simulink model "arte"  (R2013b)
(part 2 of 43)

  post_fft_delay1/3(Out2) -> antenna_power1/3(din1), [fft1_1]
  post_fft_delay1/4(Out3) -> antenna_power1/4(din2), [fft1_2]
  post_fft_delay1/5(Out4) -> antenna_power1/5(din3), [fft1_3]
  asiaa_adc5g0/12(c3) -> conv_bus1/5(i3)
  asiaa_adc5g0/14(c5) -> conv_bus1/7(i5)
  asiaa_adc5g0/10(c1) -> conv_bus1/3(i1)
  asiaa_adc5g0/13(c4) -> conv_bus1/6(i4)
  asiaa_adc5g0/9(c0) -> conv_bus1/2(i0)
  asiaa_adc5g0/15(c6) -> conv_bus1/8(i6)
  asiaa_adc5g0/16(c7) -> conv_bus1/9(i7)
  asiaa_adc5g0/11(c2) -> conv_bus1/4(i2)
  Black Box2/6 -> Terminator4/1
  bus_create2/1(bus_out) -> pipeline44/1
  pipeline44/1 -> adcsnap2/1(din)
  [cnt_rst] -> acc_cntrl2/3(rst)
  [acc_len] -> acc_cntrl2/1(acc_len)
  simple_bram_vacc_0_8/1(dout) -> pre_bram_delay2/2(In1)
  pipeline104/1(q) -> simple_bram_vacc_0_8/2(din)
  pipeline50/1(q) -> pre_bram_delay2/1(sync_in)
  pipeline49/1(q) -> simple_bram_vacc_0_8/1(new_acc)
  simple_bram_vacc_0_9/1(dout) -> pre_bram_delay2/3(In2)
  pipeline52/1(q) -> simple_bram_vacc_0_9/2(din)
  pipeline55/1(q) -> simple_bram_vacc_0_9/1(new_acc)
  simple_bram_vacc_0_10/1(dout) -> pre_bram_delay2/4(In3)
  pipeline94/1(q) -> simple_bram_vacc_0_10/2(din)
  pipeline97/1(q) -> simple_bram_vacc_0_10/1(new_acc)
  simple_bram_vacc_0_11/1(dout) -> pre_bram_delay2/5(In4)
  simple_bram_vacc_0_11/2(valid) -> pre_bram_delay2/6(valid_in)
  pipeline98/1(q) -> simple_bram_vacc_0_11/2(din)
  pipeline102/1(q) -> simple_bram_vacc_0_11/1(new_acc)
  Delay43/1 -> pipeline104/1(d)
  Delay45/1 -> pipeline52/1(d)
  Delay46/1 -> pipeline94/1(d)
  Delay47/1 -> pipeline98/1(d)
  acc_cntrl2/1(new_acc) -> pipeline102/1(d), pipeline97/1(d), pipeline55/1(d), pipeline49/1(d), pipeline50/1(d)
  Black Box3/6 -> Terminator18/1
  [cnt_rst] -> acc_cntrl3/3(rst)
  [acc_len] -> acc_cntrl3/1(acc_len)
  simple_bram_vacc_0_12/1(dout) -> pre_bram_delay3/2(In1)
  pipeline123/1(q) -> simple_bram_vacc_0_12/2(din)
  pipeline108/1(q) -> pre_bram_delay3/1(sync_in)
  pre_bram_delay3/2(Out1) -> Reinterpret12/1
  pre_bram_delay3/6(valid_out) -> Counter4/2, antenna_3/3(we)
  pre_bram_delay3/1(sync_out) -> Counter4/1
  pipeline107/1(q) -> simple_bram_vacc_0_12/1(new_acc)
  simple_bram_vacc_0_13/1(dout) -> pre_bram_delay3/3(In2)
  pipeline109/1(q) -> simple_bram_vacc_0_13/2(din)
  pre_bram_delay3/3(Out2) -> Reinterpret5/1
  pipeline112/1(q) -> simple_bram_vacc_0_13/1(new_acc)
  simple_bram_vacc_0_14/1(dout) -> pre_bram_delay3/4(In3)
  pipeline113/1(q) -> simple_bram_vacc_0_14/2(din)
  pre_bram_delay3/4(Out3) -> Reinterpret6/1
  pipeline116/1(q) -> simple_bram_vacc_0_14/1(new_acc)
  simple_bram_vacc_0_15/1(dout) -> pre_bram_delay3/5(In4)
  simple_bram_vacc_0_15/2(valid) -> pre_bram_delay3/6(valid_in)
  pipeline117/1(q) -> simple_bram_vacc_0_15/2(din)
  pre_bram_delay3/5(Out4) -> Reinterpret10/1
  pipeline120/1(q) -> simple_bram_vacc_0_15/1(new_acc)
  Delay50/1 -> pipeline123/1(d)
  Delay51/1 -> pipeline109/1(d)
  Delay52/1 -> pipeline113/1(d)
  Delay1/1 -> pipeline117/1(d)
  acc_cntrl3/1(new_acc) -> pipeline108/1(d), pipeline120/1(d), pipeline116/1(d), pipeline112/1(d), pipeline107/1(d)
  antenna_power0/2(dout0) -> power_convert0/1(In1)
  antenna_power0/3(dout1) -> power_convert0/2(In2)
  antenna_power0/4(dout2) -> power_convert0/3(In3)
  antenna_power0/5(dout3) -> power_convert0/4(In4)
  antenna_power0/1(sync_out) -> pipeline127/1(d)
  antenna_power1/2(dout0) -> power_convert1/1(In1)
  antenna_power1/3(dout1) -> power_convert1/2(In2)
  antenna_power1/4(dout2) -> power_convert1/3(In3)
  antenna_power1/5(dout3) -> power_convert1/4(In4)
  antenna_power2/2(dout0) -> power_convert2/1(In1)
  antenna_power2/3(dout1) -> power_convert2/2(In2)
  antenna_power2/4(dout2) -> power_convert2/3(In3)
  antenna_power2/5(dout3) -> power_convert2/4(In4)
  antenna_power3/2(dout0) -> power_convert3/1(In1)
  antenna_power3/3(dout1) -> power_convert3/2(In2)
  antenna_power3/4(dout2) -> power_convert3/3(In3)
  antenna_power3/5(dout3) -> power_convert3/4(In4)
  antenna_power1/1(sync_out) -> pipeline128/1(d)
  antenna_power2/1(sync_out) -> pipeline129/1(d)
  antenna_power3/1(sync_out) -> pipeline130/1(d)
  Band-Limited White Noise1/1 -> asiaa_adc5g1/1(sim_a)
  Constant2/1 -> asiaa_adc5g1/3(sim_sync)
  Band-Limited White Noise3/1 -> asiaa_adc5g1/2(sim_c)
  asiaa_adc5g1/17(sync_out) -> Terminator2/1
  asiaa_adc5g1/1(a0) -> conv_bus2/2(i0)
  asiaa_adc5g1/2(a1) -> conv_bus2/3(i1)
  asiaa_adc5g1/3(a2) -> conv_bus2/4(i2)
  asiaa_adc5g1/4(a3) -> conv_bus2/5(i3)
  asiaa_adc5g1/5(a4) -> conv_bus2/6(i4)
  asiaa_adc5g1/6(a5) -> conv_bus2/7(i5)
  asiaa_adc5g1/7(a6) -> conv_bus2/8(i6)
  asiaa_adc5g1/8(a7) -> conv_bus2/9(i7)
  asiaa_adc5g1/12(c3) -> Subsystem/4(In4)
  asiaa_adc5g1/14(c5) -> Subsystem/6(In6)
  asiaa_adc5g1/10(c1) -> Subsystem/2(In2)
  asiaa_adc5g1/13(c4) -> Subsystem/5(In5)
  asiaa_adc5g1/9(c0) -> Subsystem/1(In1)
  asiaa_adc5g1/15(c6) -> Subsystem/7(In7)
  asiaa_adc5g1/16(c7) -> Subsystem/8(In8)
  asiaa_adc5g1/11(c2) -> Subsystem/3(In3)
  [sync_out] -> delay_wideband_prog0/1(sync)
  [sync_out] -> delay_wideband_prog1/1(sync)
  [sync_out] -> delay_wideband_prog2/1(sync)
  [sync_out] -> pipeline/1(d)
  [snap_trig] -> adcsnap0/2(we), adcsnap0/3(trig)
  [snap_trig] -> adcsnap1/2(we), adcsnap1/3(trig)
  [snap_trig] -> adcsnap2/2(we), adcsnap2/3(trig)
  [adc0_delay] -> delay_wideband_prog0/2(delay)
  [adc1_delay] -> delay_wideband_prog1/2(delay)
  [adc2_delay] -> delay_wideband_prog2/2(delay)
  Constant8/1 -> delay_wideband_prog0/3(ld_delay)
  Constant9/1 -> delay_wideband_prog1/3(ld_delay)
  Constant11/1 -> delay_wideband_prog2/3(ld_delay)
  delay_wideband_prog0/9(data_out7) -> pre_pfb_delay1/9(In1)
  delay_wideband_prog0/7(data_out5) -> pre_pfb_delay1/7(In8)
  delay_wideband_prog0/2(data_out0) -> pre_pfb_delay1/2(In3)
  delay_wideband_prog0/3(data_out1) -> pre_pfb_delay1/3(In4)
  delay_wideband_prog0/5(data_out3) -> pre_pfb_delay1/5(In6)
  delay_wideband_prog0/8(data_out6) -> pre_pfb_delay1/8(In9)
  delay_wideband_prog0/4(data_out2) -> pre_pfb_delay1/4(In5)
  delay_wideband_prog0/6(data_out4) -> pre_pfb_delay1/6(In7)
  delay_wideband_prog0/1(sync_out) -> pre_pfb_delay1/1(sync_in)
  delay_wideband_prog1/1(sync_out) -> pre_pfb_delay2/1(sync_in)
  delay_wideband_prog1/2(data_out0) -> pre_pfb_delay2/2(In3)
  delay_wideband_prog1/3(data_out1) -> pre_pfb_delay2/3(In4)
  delay_wideband_prog1/4(data_out2) -> pre_pfb_delay2/4(In5)
  delay_wideband_prog1/5(data_out3) -> pre_pfb_delay2/5(In6)
  delay_wideband_prog1/6(data_out4) -> pre_pfb_delay2/6(In7)
  delay_wideband_prog1/7(data_out5) -> pre_pfb_delay2/7(In8)
  delay_wideband_prog1/8(data_out6) -> pre_pfb_delay2/8(In9)
  delay_wideband_prog1/9(data_out7) -> pre_pfb_delay2/9(In1)
  delay_wideband_prog2/1(sync_out) -> pre_pfb_delay3/1(sync_in)
  delay_wideband_prog2/2(data_out0) -> pre_pfb_delay3/2(In3)
  delay_wideband_prog2/3(data_out1) -> pre_pfb_delay3/3(In4)
  delay_wideband_prog2/4(data_out2) -> pre_pfb_delay3/4(In5)
  delay_wideband_prog2/5(data_out3) -> pre_pfb_delay3/5(In6)
  delay_wideband_prog2/6(data_out4) -> pre_pfb_delay3/6(In7)
  delay_wideband_prog2/7(data_out5) -> pre_pfb_delay3/7(In8)
  delay_wideband_prog2/8(data_out6) -> pre_pfb_delay3/8(In9)
  delay_wideband_prog2/9(data_out7) -> pre_pfb_delay3/9(In1)
  conv_bus4/1(q0) -> delay_wideband_prog0/4(data_in0)
  conv_bus4/2(q1) -> delay_wideband_prog0/5(data_in1)
  conv_bus4/3(q2) -> delay_wideband_prog0/6(data_in2)
  conv_bus4/4(q3) -> delay_wideband_prog0/7(data_in3)
  conv_bus4/5(q4) -> delay_wideband_prog0/8(data_in4)
  conv_bus4/6(q5) -> delay_wideband_prog0/9(data_in5)
  conv_bus4/7(q6) -> delay_wideband_prog0/10(data_in6)
  conv_bus4/8(q7) -> delay_wideband_prog0/11(data_in7)
  conv_bus1/1(q0) -> delay_wideband_prog1/4(data_in0)
  conv_bus1/2(q1) -> delay_wideband_prog1/5(data_in1)
  conv_bus1/3(q2) -> delay_wideband_prog1/6(data_in2)
  conv_bus1/4(q3) -> delay_wideband_prog1/7(data_in3)
  conv_bus1/5(q4) -> delay_wideband_prog1/8(data_in4)
  conv_bus1/6(q5) -> delay_wideband_prog1/9(data_in5)
  conv_bus1/7(q6) -> delay_wideband_prog1/10(data_in6)
  conv_bus1/8(q7) -> delay_wideband_prog1/11(data_in7)
  conv_bus2/1(q0) -> delay_wideband_prog2/4(data_in0)
  conv_bus2/2(q1) -> delay_wideband_prog2/5(data_in1)
  conv_bus2/3(q2) -> delay_wideband_prog2/6(data_in2)
  conv_bus2/4(q3) -> delay_wideband_prog2/7(data_in3)
  conv_bus2/5(q4) -> delay_wideband_prog2/8(data_in4)
  conv_bus2/6(q5) -> delay_wideband_prog2/9(data_in5)
  conv_bus2/7(q6) -> delay_wideband_prog2/10(data_in6)
  conv_bus2/8(q7) -> delay_wideband_prog2/11(data_in7)
  pre_pfb_delay1/2(Out3) -> bus_create/1(in1), Black Box6/2
  pre_pfb_delay1/3(Out4) -> bus_create/2(in2), Black Box6/3
  pre_pfb_delay1/4(Out5) -> Black Box6/4, bus_create/3(in3)
  pre_pfb_delay1/5(Out6) -> Black Box6/5, bus_create/4(in4)
  pre_pfb_delay1/6(Out7) -> bus_create/5(in5), Black Box6/6
  pre_pfb_delay1/7(Out8) -> Black Box6/7, bus_create/6(in6)
  pre_pfb_delay1/8(Out9) -> bus_create/7(in7), Black Box6/8
  pre_pfb_delay1/9(Out1) -> Black Box6/9, bus_create/8(in8)
  pre_pfb_delay2/9(Out1) -> Black Box1/9, bus_create1/8(in8)
  pre_pfb_delay2/2(Out3) -> Black Box1/2, bus_create1/1(in1)
  pre_pfb_delay2/3(Out4) -> bus_create1/2(in2), Black Box1/3
  pre_pfb_delay2/8(Out9) -> bus_create1/7(in7), Black Box1/8
  pre_pfb_delay2/7(Out8) -> Black Box1/7, bus_create1/6(in6)
  pre_pfb_delay2/6(Out7) -> Black Box1/6, bus_create1/5(in5)
  pre_pfb_delay2/5(Out6) -> bus_create1/4(in4), Black Box1/5
  pre_pfb_delay2/4(Out5) -> Black Box1/4, bus_create1/3(in3)
  pre_pfb_delay3/9(Out1) -> Black Box2/9, bus_create2/8(in8)
  pre_pfb_delay3/8(Out9) -> Black Box2/8, bus_create2/7(in7)
  pre_pfb_delay3/7(Out8) -> bus_create2/6(in6), Black Box2/7
  pre_pfb_delay3/6(Out7) -> Black Box2/6, bus_create2/5(in5)
  pre_pfb_delay3/5(Out6) -> Black Box2/5, bus_create2/4(in4)
  pre_pfb_delay3/4(Out5) -> bus_create2/3(in3), Black Box2/4
  pre_pfb_delay3/3(Out4) -> Black Box2/3, bus_create2/2(in2)
  pre_pfb_delay3/2(Out3) -> Black Box2/2, bus_create2/1(in1)
  pipeline/1(q) -> delay_pre_pfb/1
  pre_pfb_delay1/1(sync_out) -> Black Box6/1
  pre_pfb_delay2/1(sync_out) -> Black Box1/1
  pre_pfb_delay3/1(sync_out) -> Black Box2/1
  delay_pre_pfb/1 -> Black Box3/1
  Black Box6/5 -> post_fft_delay0/5(In4)
  Black Box6/3 -> post_fft_delay0/3(In2)
  Black Box6/4 -> post_fft_delay0/4(In3)
  Black Box6/2 -> post_fft_delay0/2(In1)
  Black Box6/1 -> post_fft_delay0/1(sync_in)
  Black Box1/5 -> post_fft_delay1/5(In4)
  Black Box1/3 -> post_fft_delay1/3(In2)
  Black Box1/2 -> post_fft_delay1/2(In1)
  Black Box1/4 -> post_fft_delay1/4(In3)
  Black Box1/1 -> post_fft_delay1/1(sync_in)
  Black Box2/5 -> post_fft_delay2/5(In4)
  Black Box2/1 -> post_fft_delay2/1(sync_in)
  Black Box2/2 -> post_fft_delay2/2(In1)
  Black Box2/4 -> post_fft_delay2/4(In3)
  Black Box2/3 -> post_fft_delay2/3(In2)
  Black Box3/4 -> post_fft_delay3/4(In3)
  Black Box3/2 -> post_fft_delay3/2(In1)
  Black Box3/5 -> post_fft_delay3/5(In4)
  Black Box3/3 -> post_fft_delay3/3(In2)
  Black Box3/1 -> post_fft_delay3/1(sync_in)
  bus_create3/1(bus_out) -> pipeline6/1
  pipeline6/1 -> adcsnap3/1(din)
  [snap_trig] -> adcsnap3/2(we), adcsnap3/3(trig)
  Subsystem/8(Out8) -> bus_create3/8(in8), Black Box3/9
  Subsystem/7(Out7) -> bus_create3/7(in7), Black Box3/8
  Subsystem/6(Out6) -> bus_create3/6(in6), Black Box3/7
  Subsystem/5(Out5) -> bus_create3/5(in5), Black Box3/6
  Subsystem/4(Out4) -> bus_create3/4(in4), Black Box3/5
  Subsystem/3(Out3) -> bus_create3/3(in3), Black Box3/4
  Subsystem/2(Out2) -> bus_create3/2(in2), Black Box3/3
  Subsystem/1(Out1) -> bus_create3/1(in1), Black Box3/2
  post_fft_delay2/1(sync_out) -> antenna_power2/1(sync_in), [sync_out2]
  post_fft_delay2/2(Out1) -> antenna_power2/2(din0), [fft2_0]
  post_fft_delay2/3(Out2) -> antenna_power2/3(din1), [fft2_1]
  post_fft_delay2/4(Out3) -> antenna_power2/4(din2), [fft2_2]
  post_fft_delay2/5(Out4) -> antenna_power2/5(din3), [fft2_3]
  post_fft_delay3/1(sync_out) -> antenna_power3/1(sync_in), [sync_out3]
  post_fft_delay3/2(Out1) -> antenna_power3/2(din0), [fft3_0]
  post_fft_delay3/3(Out2) -> antenna_power3/3(din1), [fft3_1]
  post_fft_delay3/4(Out3) -> antenna_power3/4(din2), [fft3_2]
  post_fft_delay3/5(Out4) -> antenna_power3/5(din3), [fft3_3]
  pipeline127/1(q) -> acc_cntrl0/2(sync)
  power_convert0/1(Out1) -> Delay32/1
  power_convert0/2(Out2) -> Delay34/1
  power_convert0/3(Out3) -> Delay35/1
  power_convert0/4(Out4) -> Delay36/1
  pipeline128/1(q) -> acc_cntrl1/2(sync)
  power_convert1/1(Out1) -> Delay7/1
  power_convert1/2(Out2) -> Delay8/1
  power_convert1/3(Out3) -> Delay9/1
  power_convert1/4(Out4) -> Delay10/1
  pipeline129/1(q) -> acc_cntrl2/2(sync)
  power_convert2/1(Out1) -> Delay43/1
  power_convert2/2(Out2) -> Delay45/1
  power_convert2/3(Out3) -> Delay46/1
  power_convert2/4(Out4) -> Delay47/1
  pipeline130/1(q) -> acc_cntrl3/2(sync)
  power_convert3/1(Out1) -> Delay50/1
  power_convert3/2(Out2) -> Delay51/1
  power_convert3/3(Out3) -> Delay52/1
  power_convert3/4(Out4) -> Delay1/1
  Concat/1 -> antenna_0/2(data_in)
  Counter1/1 -> antenna_0/1(addr)
  Concat1/1 -> antenna_1/2(data_in)
  Counter2/1 -> antenna_1/1(addr)
  Concat2/1 -> antenna_2/2(data_in)
  Counter3/1 -> antenna_2/1(addr)
  Concat3/1 -> antenna_3/2(data_in)
  Counter4/1 -> antenna_3/1(addr)
  simple_bram_vacc_0_0/1(dout) -> pre_bram_delay0/2(In1)
  simple_bram_vacc_0_1/1(dout) -> pre_bram_delay0/3(In2)
  simple_bram_vacc_0_2/1(dout) -> pre_bram_delay0/4(In3)
  simple_bram_vacc_0_3/1(dout) -> pre_bram_delay0/5(In4)
  simple_bram_vacc_0_3/2(valid) -> pre_bram_delay0/6(valid_in)
  pipeline59/1(q) -> pre_bram_delay0/1(sync_in)
  pipeline77/1(q) -> pre_bram_delay1/1(sync_in)
  pre_bram_delay2/1(sync_out) -> Counter3/1
  pre_bram_delay2/2(Out1) -> Reinterpret11/1
  pre_bram_delay2/3(Out2) -> Reinterpret7/1
  pre_bram_delay2/4(Out3) -> Reinterpret8/1
  pre_bram_delay2/5(Out4) -> Reinterpret9/1
  pre_bram_delay2/6(valid_out) -> Counter3/2, antenna_2/3(we)
  control/1(cnt_rst) -> [cnt_rst]
  control/2(snap_trig) -> [snap_trig]
  control/3(adc0_delay) -> [adc0_delay]
  control/4(adc1_delay) -> [adc1_delay]
  control/5(adc2_delay) -> [adc2_delay]
  control/6(adc3_delay) -> [adc3_delay]
  control/7(gbe_ip) -> [gbe_ip]
  control/8(gbe_port) -> [gbe_port]
  control/9(tge_ip) -> [tge_ip]
  control/10(tge_port) -> [tge_port]
  control/11(adc_gain) -> [adc_gain]
  control/12(rst_detection) -> [rst_detection]
  [adc_gain] -> conv_bus4/1(gain)
  [adc_gain] -> conv_bus1/1(gain)
  [adc_gain] -> conv_bus2/1(gain)
  conv_bus4/9(reduced) -> [adc0]
  conv_bus1/9(reduced) -> [adc1]
  conv_bus2/9(reduced) -> [adc2]
  [fft0_0] -> complex_add/1(ff0_ch0)
  [fft1_0] -> complex_add/2(fft1_ch0)
  [fft0_1] -> complex_add/3(fft0_ch1)
  [fft1_1] -> complex_add/4(fft1_ch1)
  [fft0_2] -> complex_add/5(fft0_ch2)
  [fft1_2] -> complex_add/6(fft1_ch2)
  [fft0_3] -> complex_add/7(fft0_ch3)
  [fft1_3] -> complex_add/8(fft1_ch3)
  [sync_out0] -> complex_add/9(sync)
  complex_add/3(ch1) -> beam_post_complex_add/3(In2)
  complex_add/1(sync_out) -> beam_post_complex_add/1(sync_in)
  complex_add/2(ch0) -> beam_post_complex_add/2(In1)
  complex_add/5(ch3) -> beam_post_complex_add/5(In4)
  complex_add/4(ch2) -> beam_post_complex_add/4(In3)
  beam_post_complex_add/5(Out4) -> concat_order/4(ch3), beam_power/5(din3)
  beam_post_complex_add/4(Out3) -> beam_power/4(din2), concat_order/3(ch2)
  beam_post_complex_add/3(Out2) -> concat_order/2(ch1), beam_power/3(din1)
  beam_post_complex_add/2(Out1) -> concat_order/1(ch0), beam_power/2(din0)
  beam_power/1(sync_out) -> post_flag_delay1/1(sync_in)
  [cnt_rst] -> acc_cntrl4/3(rst)
  [acc_len] -> acc_cntrl4/1(acc_len)
  pipeline11/1(q) -> beam_vacc0/2(din)
  pipeline1/1(q) -> beam_vacc0/1(new_acc)
  pipeline3/1(q) -> beam_vacc1/2(din)
  pipeline5/1(q) -> beam_vacc1/1(new_acc)
  pipeline7/1(q) -> beam_vacc2/2(din)
  pipeline8/1(q) -> beam_vacc2/1(new_acc)
  pipeline9/1(q) -> beam_vacc3/2(din)
  pipeline10/1(q) -> beam_vacc3/1(new_acc)
  Delay2/1 -> pipeline11/1(d)
  Delay3/1 -> pipeline3/1(d)
  Delay4/1 -> pipeline7/1(d)
  Delay5/1 -> pipeline9/1(d)
  acc_cntrl4/1(new_acc) -> pipeline10/1(d), pipeline8/1(d), pipeline5/1(d), pipeline1/1(d), pipeline2/1(d)
  beam_power_conv/1(sync_out) -> acc_cntrl4/2(sync)
  beam_power_conv/2(Out1) -> Delay2/1
  beam_power_conv/3(Out2) -> Delay3/1
  beam_power_conv/4(Out3) -> Delay4/1
  beam_power_conv/5(Out4) -> Delay5/1
  Concat4/1 -> beam/2(data_in)
  Counter5/1 -> beam/1(addr)
  beam_vacc0/1(dout) -> beam_post_acc_delay/2(In1)
  beam_vacc1/1(dout) -> beam_post_acc_delay/3(In2)
  beam_vacc2/1(dout) -> beam_post_acc_delay/4(In3)
  beam_vacc3/1(dout) -> beam_post_acc_delay/5(In4)
  beam_vacc3/2(valid) -> beam_post_acc_delay/6(valid_in)
  pipeline2/1(q) -> beam_post_acc_delay/1(sync_in)
  concat_/1(Out1) -> Mux/2
  beam_post_acc_delay/6(valid_out) -> pipeline23/1(d), Counter5/2, beam/3(we)
  Logical/1 -> pipeline12/1(d)
  Register/1 -> Logical1/1
  pipeline12/1(q) -> Logical1/2
  Inverter/1 -> Register/2
  [tge_en] -> Inverter/1
  Constant6/1 -> ten_Gbe_v2/7
  ten_Gbe_v2/12 -> Delay/1
  Delay/1 -> ten_Gbe_v2/8
  ten_Gbe_v2/1 -> Terminator14/1
  ten_Gbe_v2/2 -> Terminator15/1
  ten_Gbe_v2/3 -> gpio1/1
  ten_Gbe_v2/4 -> Terminator3/1
  ten_Gbe_v2/5 -> Terminator19/1
  ten_Gbe_v2/6 -> Terminator20/1
  ten_Gbe_v2/7 -> Terminator21/1
  ten_Gbe_v2/8 -> Terminator22/1
  ten_Gbe_v2/9 -> Terminator23/1
  ten_Gbe_v2/10 -> Terminator24/1
  ten_Gbe_v2/11 -> Terminator25/1
  ten_Gbe_v2/13 -> Terminator26/1
  ten_Gbe_v2/14 -> Terminator27/1
  [tge_rst] -> ten_Gbe_v2/1
  pipeline19/1(q) -> concat_/1(In1)
  pipeline20/1(q) -> concat_/2(In2)
  pipeline21/1(q) -> concat_/3(In3)
  pipeline22/1(q) -> concat_/4(In4)
  pipeline23/1(q) -> Logical/2
  [tge_rst] -> Register1/2
  Register1/1 -> gpio/1
  Convert/1 -> Register1/3, Register1/1
  beam_post_acc_delay/2(Out1) -> pipeline19/1(d), Reinterpret16/1
  beam_post_acc_delay/5(Out4) -> pipeline22/1(d), Reinterpret15/1
  beam_post_acc_delay/4(Out3) -> pipeline21/1(d), Reinterpret14/1
  beam_post_acc_delay/3(Out2) -> pipeline20/1(d), Reinterpret13/1
  beam_post_acc_delay/1(sync_out) -> pipeline18/1(d), Counter5/1
  pipeline18/1(q) -> Mux/1, Register/3, Register/1, Logical/1
  [header] -> Mux/3
  control/13(tge_pkt) -> [tge_pkt]
  control/14(tge_sleep) -> [tge_sleep]
  control/15(tge_en) -> [tge_en]
  Constant/1 -> Concat5/1
  Constant1/1 -> Concat5/2
  Constant3/1 -> Concat5/3
  Constant5/1 -> Concat5/4
  Concat5/1 -> [header]
  [rst] -> pipeline421/1
  [rst] -> pipeline422/1
  [gbe_data] -> pipeline423/1
  [gbe_valid] -> pipeline424/1
  [gbe_eof] -> pipeline430/1
  Delay91/1 -> pipeline428/1
  one_GbE/1 -> Terminator59/1
  one_GbE/2 -> Terminator60/1
  one_GbE/3 -> Terminator61/1
  one_GbE/4 -> Terminator53/1
  one_GbE/5 -> Terminator54/1
  one_GbE/6 -> Terminator55/1
  one_GbE/7 -> Terminator56/1
  one_GbE/8 -> Terminator57/1
  one_GbE/9 -> Terminator58/1
  one_GbE/10 -> Terminator51/1
  one_GbE/11 -> Terminator52/1
  Concat6/1 -> pipeline406/1(d)
  ring/1(dout) -> pipeline403/1
  ring/2(eof) -> pipeline404/1
  ring/3(val) -> pipeline405/1
  pipeline407/1 -> Concat6/1
  pipeline408/1 -> Concat6/2
  pipeline409/1 -> Concat6/3
  pipeline406/1(q) -> ring/2(data_in)
  [adc0] -> pipeline407/1
  [adc1] -> pipeline408/1
  [adc2] -> pipeline409/1
  [gbe_port] -> Delay92/1
  [gbe_ip] -> Delay91/1
  control1/1(in_reg) -> Slice12/1, Slice11/1, Slice10/1
  Slice10/1 -> Delay6/1
  Slice11/1 -> Delay49/1
  Delay6/1 -> [write]
  Delay49/1 -> [rst]
  Slice12/1 -> Delay11/1
  Delay11/1 -> [allow_detect]
  [detection] -> Delay93/1
  [write] -> Logical24/2
  Logical23/1 -> Logical24/1
  [allow_detect] -> Inverter3/1
  Logical24/1 -> gpio2/1, ring/1(write_en)
  Inverter3/1 -> Logical23/1
  pipeline403/1 -> [gbe_data]
  pipeline404/1 -> [gbe_eof]
  pipeline405/1 -> [gbe_valid]
  Delay93/1 -> Logical23/2
  pipeline421/1 -> one_GbE/1
  pipeline422/1 -> one_GbE/2
  pipeline423/1 -> one_GbE/3
  pipeline424/1 -> one_GbE/4
  pipeline428/1 -> one_GbE/5
  pipeline429/1 -> one_GbE/6
  pipeline430/1 -> one_GbE/7
  Delay92/1 -> pipeline429/1
  Constant105/1 -> one_GbE/8
  Logical3/1 -> [detection], gpio3/1
  control/16(rst_tge) -> [tge_rst]
  beam_post_complex_add/1(sync_out) -> beam_power/1(sync_in), Black Box5/1
  concat_order/1(Out1) -> Black Box5/2
  [flag_rfi] -> Black Box5/3
  [flag_num] -> Black Box5/4
  [flag_en] -> Black Box5/5
  Counter6/1 -> Slice8/1, Slice7/1, Slice6/1
  Slice6/1 -> Logical2/2
  Slice7/1 -> Logical2/3
  Subsystem3/1(Out1) -> pre_dedisp_acc_conv/2(din)
  Slice8/1 -> Logical2/1
  Logical2/1 -> pre_dedisp_acc_conv/3(din_valid)
  adder_tree1/1(sync_out) -> pre_dedisp_acc_conv/1(sync_in), Counter6/1
  adder_tree1/2(dout) -> Subsystem3/1(In1)
  Black Box5/2 -> Slice9/1, Slice2/1, Slice5/1, Slice3/1, Slice1/1, Slice4/1, Slice16/1, Slice17/1
  Black Box5/1 -> Convert5/1, Convert46/1
  Convert46/1 -> post_flag_delay/1(sync_in)
  Slice4/1 -> post_flag_delay/2(In1)
  Slice9/1 -> post_flag_delay/3(In2)
  Slice16/1 -> post_flag_delay/4(In3)
  Slice17/1 -> post_flag_delay/5(In4)
  post_flag_delay/2(Out1) -> flag_power/2(din0)
  post_flag_delay/4(Out3) -> flag_power/4(din2)
  post_flag_delay/3(Out2) -> flag_power/3(din1)
  post_flag_delay/1(sync_out) -> flag_power/1(sync_in)
  post_flag_delay/5(Out4) -> flag_power/5(din3)
  flag_power/5(dout3) -> flag_convert/5(In4)
  flag_power/1(sync_out) -> flag_convert/1(sync_in)
  flag_power/4(dout2) -> flag_convert/4(In3)
  flag_power/2(dout0) -> flag_convert/2(In1)
  flag_power/3(dout1) -> flag_convert/3(In2)
  flag_convert/1(sync_out) -> adder_tree1/1(sync)
  flag_convert/3(Out2) -> adder_tree1/3(din2)
  flag_convert/5(Out4) -> adder_tree1/5(din4)
  flag_convert/2(Out1) -> adder_tree1/2(din1)
  flag_convert/4(Out3) -> adder_tree1/4(din3)
  control/17(flag_en) -> [flag_en]
  control/18(flag_num) -> [flag_num]
  control/19(flag_rfi) -> [flag_rfi]
  control/20(acc_len0) -> [acc_len]
  control/21(acc_len1) -> [acc_len0]
  control/22(acc_len2) -> [acc_len1]
  control/23(acc_len3) -> [acc_len2]
  control/24(acc_len4) -> [acc_len3]
  Reinterpret31/1 -> Concat/1
  Reinterpret24/1 -> Concat/2
  Reinterpret25/1 -> Concat/3
  Reinterpret26/1 -> Concat/4
  Reinterpret4/1 -> Concat1/1
  Reinterpret1/1 -> Concat1/2
  Reinterpret2/1 -> Concat1/3
  Reinterpret3/1 -> Concat1/4
  Reinterpret11/1 -> Concat2/1
  Reinterpret7/1 -> Concat2/2
  Reinterpret8/1 -> Concat2/3
  Reinterpret9/1 -> Concat2/4
  Reinterpret12/1 -> Concat3/1
  Reinterpret5/1 -> Concat3/2
  Reinterpret6/1 -> Concat3/3
  Reinterpret10/1 -> Concat3/4
  Reinterpret16/1 -> Concat4/1
  Reinterpret13/1 -> Concat4/2
  Reinterpret14/1 -> Concat4/3
  Reinterpret15/1 -> Concat4/4
  pipeline30/1 -> sync_tree2/1(In1)
  pipeline53/1 -> m0_tree2/1(In1)
  pipeline27/1 -> m0_en1/1(In1)
  pre_dedisp_acc_conv/2(dout) -> pipeline53/1
  pre_dedisp_acc_conv/1(sync_out) -> pipeline30/1
  pre_dedisp_acc_conv/3(dout_valid) -> pipeline27/1
  control/32(rst_dedisp) -> [rst_dedisp]
  control/34(theta1) -> [theta0]
  control/35(theta2) -> [theta1]
  control/36(theta3) -> [theta2]
  control/37(theta4) -> [theta3]
  [acc_len0] -> acc_cntrl5/1(acc_len)
  [sd0] -> acc_cntrl5/2(sync)
  [cnt_rst] -> acc_cntrl5/3(rst)
  Logical27/1 -> enabled_vacc0/1(new_acc), pipeline24/1(d), Register16/3, Register16/1
  pipeline15/1(q) -> enabled_vacc0/2(din)
  [m0e0] -> pipeline16/1(d)
  [m0d0] -> pipeline15/1(d)
  enabled_vacc0/1(dout) -> Convert2/1, pre_dedisp_conv0/1(din)
  enabled_vacc0/2(dout_valid) -> pipeline17/1(d), pre_dedisp_conv0/2(din_valid)
  pre_dedisp_conv0/2(dout_valid) -> pre_dedisp_delay0/2(din_valid)
  pre_dedisp_conv0/1(dout) -> pre_dedisp_delay0/1(In1)
  pre_dedisp_delay0/2(dout_valid) -> dedispersor0/3(din_valid)
  pre_dedisp_delay0/1(Out1) -> dedispersor0/2(din)
  [rst_dedisp] -> dedispersor0/1(rst)
  dedispersor0/1(integ_pow) -> post_dedisp_conv0/1(din)
  dedispersor0/2(integ_valid) -> post_dedisp_conv0/2(din_valid)
  post_dedisp_conv0/1(dout) -> post_dedisp_delay0/1(In1)
  post_dedisp_conv0/2(dout_valid) -> post_dedisp_delay0/2(din_valid)
  post_dedisp_delay0/1(Out1) -> Convert3/1, Relational/1, mov_avg0/2(din)
  [rst_dedisp] -> mov_avg0/1(rst)
  mov_avg0/1(dout) -> add_stat0/2
  add_stat0/1 -> Relational/2, Convert4/1
  [theta0] -> add_stat0/1
  Logical11/1 -> pipeline42/1
  [rst_detection] -> Register2/2
  Register2/1 -> [detection0]
  Convert2/1 -> Reinterpret17/1
  Reinterpret17/1 -> debug_acc/2(data_in)
  pipeline24/1(q) -> Counter7/1
  pipeline17/1(q) -> Counter7/2, debug_acc/3(we)
  Counter7/1 -> debug_acc/1(addr)
  Counter8/1 -> dedisp0/1(addr)
  post_dedisp_delay0/2(dout_valid) -> Counter8/1, dedisp0/3(we), mov_avg0/3(din_valid)
  Convert3/1 -> Reinterpret19/1
  Reinterpret19/1 -> dedisp0/2(data_in)
  Counter9/1 -> avg0/1(addr)
  mov_avg0/2(dout_valid) -> Counter9/1, avg0/3(we)
  Convert4/1 -> Reinterpret20/1
  Reinterpret20/1 -> avg0/2(data_in)
  Convert5/1 -> beam_rfi_delay/1(sync_in)
  Slice3/1 -> beam_rfi_delay/2(In1)
  Slice5/1 -> beam_rfi_delay/3(In2)
  Slice1/1 -> beam_rfi_delay/4(In3)
  Slice2/1 -> beam_rfi_delay/5(In4)
  beam_rfi_delay/1(sync_out) -> [beam_sync]
  beam_rfi_delay/2(Out1) -> [beam0]
  beam_rfi_delay/3(Out2) -> [beam1]
  beam_rfi_delay/4(Out3) -> [beam2]
  beam_rfi_delay/5(Out4) -> [beam3]
  [sync_out3] -> rfi_delay/1(sync_in)
  [fft3_0] -> rfi_delay/2(In1)
  [fft3_1] -> rfi_delay/3(In2)
  [fft3_2] -> rfi_delay/4(In3)
  [fft3_3] -> rfi_delay/5(In4)
  rfi_delay/1(sync_out) -> [rfi_sync]
  rfi_delay/2(Out1) -> [rfi0]
  rfi_delay/3(Out2) -> [rfi1]
  rfi_delay/4(Out3) -> [rfi2]
  rfi_delay/5(Out4) -> [rfi3]
  [tge_rst] -> packetizer/1(rst)
  Mux/1 -> packetizer/2(din)
  [tge_pkt] -> packetizer/3(pkt_len)
  [tge_sleep] -> packetizer/4(sleep_cycle)
  [tge_ip] -> packetizer/5(config_tx_dest_ip)
  Logical1/1 -> packetizer/6(din_valid)
  [tge_port] -> packetizer/7(config_tx_dest_port)
  packetizer/1(tx_data) -> ten_Gbe_v2/2
  packetizer/2(tx_valid) -> ten_Gbe_v2/3
  packetizer/3(tx_dest_ip) -> ten_Gbe_v2/4
  packetizer/4(tx_dest_port) -> ten_Gbe_v2/5
  packetizer/5(tx_eof) -> ten_Gbe_v2/6
  packetizer/6(fifo_full) -> Convert/1
  [acc_len1] -> acc_cntrl6/1(acc_len)
  [sd0] -> acc_cntrl6/2(sync)
  [cnt_rst] -> acc_cntrl6/3(rst)
  pipeline33/1(q) -> enabled_vacc1/2(din)
  [m0e1] -> pipeline34/1(d)
  [m0d1] -> pipeline33/1(d)
  enabled_vacc1/1(dout) -> pre_dedisp_conv1/1(din)
  enabled_vacc1/2(dout_valid) -> pre_dedisp_conv1/2(din_valid)
  pre_dedisp_conv1/2(dout_valid) -> pre_dedisp_delay1/2(din_valid)
  pre_dedisp_conv1/1(dout) -> pre_dedisp_delay1/1(In1)
  pre_dedisp_delay1/2(dout_valid) -> dedispersor1/3(din_valid)
  pre_dedisp_delay1/1(Out1) -> dedispersor1/2(din)
  [rst_dedisp] -> dedispersor1/1(rst)
  dedispersor1/1(integ_pow) -> post_dedisp_conv1/1(din)
  dedispersor1/2(integ_valid) -> post_dedisp_conv1/2(din_valid)
  post_dedisp_conv1/1(dout) -> post_dedisp_delay1/1(In1)
  post_dedisp_conv1/2(dout_valid) -> post_dedisp_delay1/2(din_valid)
  post_dedisp_delay1/1(Out1) -> Convert7/1, Relational1/1, mov_avg1/2(din)
  [rst_dedisp] -> mov_avg1/1(rst)
  mov_avg1/1(dout) -> add_stat1/2
  add_stat1/1 -> Relational1/2, Convert8/1
  [theta1] -> add_stat1/1
  [rst_detection] -> Register3/2
  Register3/1 -> [detection1]
  Counter13/1 -> dedisp1/1(addr)
  post_dedisp_delay1/2(dout_valid) -> Counter13/1, dedisp1/3(we), mov_avg1/3(din_valid)
  Convert7/1 -> Reinterpret35/1
  Reinterpret35/1 -> dedisp1/2(data_in)
  Counter14/1 -> avg1/1(addr)
  mov_avg1/2(dout_valid) -> Counter14/1, avg1/3(we)
  Convert8/1 -> Reinterpret36/1
  Reinterpret36/1 -> avg1/2(data_in)
  [acc_len2] -> acc_cntrl7/1(acc_len)
  [sd0] -> acc_cntrl7/2(sync)
  [cnt_rst] -> acc_cntrl7/3(rst)
  pipeline35/1(q) -> enabled_vacc2/2(din)
  [m0e2] -> pipeline36/1(d)
  [m0d2] -> pipeline35/1(d)
  enabled_vacc2/1(dout) -> pre_dedisp_conv2/1(din)
  enabled_vacc2/2(dout_valid) -> pre_dedisp_conv2/2(din_valid)
  pre_dedisp_conv2/2(dout_valid) -> pre_dedisp_delay2/2(din_valid)
  pre_dedisp_conv2/1(dout) -> pre_dedisp_delay2/1(In1)
  pre_dedisp_delay2/2(dout_valid) -> dedispersor2/3(din_valid)
  pre_dedisp_delay2/1(Out1) -> dedispersor2/2(din)
  [rst_dedisp] -> dedispersor2/1(rst)
  dedispersor2/1(integ_pow) -> post_dedisp_conv2/1(din)
  dedispersor2/2(integ_valid) -> post_dedisp_conv2/2(din_valid)
  post_dedisp_conv2/1(dout) -> post_dedisp_delay2/1(In1)
  post_dedisp_conv2/2(dout_valid) -> post_dedisp_delay2/2(din_valid)
  post_dedisp_delay2/1(Out1) -> Convert6/1, Relational2/1, mov_avg2/2(din)
  [rst_dedisp] -> mov_avg2/1(rst)
  mov_avg2/1(dout) -> add_stat2/2
  add_stat2/1 -> Relational2/2, Convert9/1
  [theta2] -> add_stat2/1
  [rst_detection] -> Register4/2
  Register4/1 -> [detection2]
  Counter12/1 -> dedisp2/1(addr)
  post_dedisp_delay2/2(dout_valid) -> Counter12/1, dedisp2/3(we), mov_avg2/3(din_valid)
  Convert6/1 -> Reinterpret37/1
  Reinterpret37/1 -> dedisp2/2(data_in)
  Counter15/1 -> avg2/1(addr)
  mov_avg2/2(dout_valid) -> Counter15/1, avg2/3(we)
  Convert9/1 -> Reinterpret38/1
  Reinterpret38/1 -> avg2/2(data_in)
  [acc_len3] -> acc_cntrl8/1(acc_len)
  [sd0] -> acc_cntrl8/2(sync)
  [cnt_rst] -> acc_cntrl8/3(rst)
  pipeline37/1(q) -> enabled_vacc3/2(din)
  [m0e3] -> pipeline38/1(d)
  [m0d3] -> pipeline37/1(d)
  enabled_vacc3/1(dout) -> pre_dedisp_conv3/1(din)
  enabled_vacc3/2(dout_valid) -> pre_dedisp_conv3/2(din_valid)
  pre_dedisp_conv3/2(dout_valid) -> pre_dedisp_delay3/2(din_valid)
  pre_dedisp_conv3/1(dout) -> pre_dedisp_delay3/1(In1)
  pre_dedisp_delay3/2(dout_valid) -> dedispersor3/3(din_valid)
  pre_dedisp_delay3/1(Out1) -> dedispersor3/2(din)
  [rst_dedisp] -> dedispersor3/1(rst)
  dedispersor3/1(integ_pow) -> post_dedisp_conv3/1(din)
  dedispersor3/2(integ_valid) -> post_dedisp_conv3/2(din_valid)
  post_dedisp_conv3/1(dout) -> post_dedisp_delay3/1(In1)
  post_dedisp_conv3/2(dout_valid) -> post_dedisp_delay3/2(din_valid)
  post_dedisp_delay3/1(Out1) -> Convert10/1, Relational3/1, mov_avg3/2(din)
  [rst_dedisp] -> mov_avg3/1(rst)
  mov_avg3/1(dout) -> add_stat3/2
  add_stat3/1 -> Relational3/2, Convert11/1
  [theta3] -> add_stat3/1
  [rst_detection] -> Register5/2
  Register5/1 -> [detection3]
  Counter16/1 -> dedisp3/1(addr)
  post_dedisp_delay3/2(dout_valid) -> Counter16/1, dedisp3/3(we), mov_avg3/3(din_valid)
  Convert10/1 -> Reinterpret40/1
  Reinterpret40/1 -> dedisp3/2(data_in)
  Counter17/1 -> avg3/1(addr)
  mov_avg3/2(dout_valid) -> Counter17/1, avg3/3(we)
  Convert11/1 -> Reinterpret41/1
  Reinterpret41/1 -> avg3/2(data_in)
  [detection0] -> Logical3/1
  [detection1] -> Logical3/2
  [detection2] -> Logical3/3
  [detection3] -> Logical3/4
  pipeline39/1 -> Register5/3, Register5/1
  pipeline40/1 -> Register4/3, Register4/1
  pipeline41/1 -> Register3/3, Register3/1
  pipeline42/1 -> Register2/3, Register2/1
  [acc_len4] -> acc_cntrl9/1(acc_len)
  [sd0] -> acc_cntrl9/2(sync)
  [cnt_rst] -> acc_cntrl9/3(rst)
  pipeline43/1(q) -> enabled_vacc4/2(din)
  [m0e4] -> pipeline45/1(d)
  [m0d4] -> pipeline43/1(d)
  enabled_vacc4/1(dout) -> pre_dedisp_conv4/1(din)
  enabled_vacc4/2(dout_valid) -> pre_dedisp_conv4/2(din_valid)
  pre_dedisp_conv4/2(dout_valid) -> pre_dedisp_delay4/2(din_valid)
  pre_dedisp_conv4/1(dout) -> pre_dedisp_delay4/1(In1)
  pre_dedisp_delay4/2(dout_valid) -> dedispersor4/3(din_valid)
  pre_dedisp_delay4/1(Out1) -> dedispersor4/2(din)
  [rst_dedisp] -> dedispersor4/1(rst)
  dedispersor4/1(integ_pow) -> post_dedisp_conv4/1(din)
  dedispersor4/2(integ_valid) -> post_dedisp_conv4/2(din_valid)
  post_dedisp_conv4/1(dout) -> post_dedisp_delay4/1(In1)
  post_dedisp_conv4/2(dout_valid) -> post_dedisp_delay4/2(din_valid)
  post_dedisp_delay4/1(Out1) -> Convert12/1, Relational4/1, mov_avg4/2(din)
  [rst_dedisp] -> mov_avg4/1(rst)
  mov_avg4/1(dout) -> add_stat4/2
  add_stat4/1 -> Relational4/2, Convert13/1
  [theta4] -> add_stat4/1
  [rst_detection] -> Register6/2
  Register6/1 -> [detection4]
  Counter18/1 -> dedisp4/1(addr)
  post_dedisp_delay4/2(dout_valid) -> Counter18/1, dedisp4/3(we), mov_avg4/3(din_valid)
  Convert12/1 -> Reinterpret43/1
  Reinterpret43/1 -> dedisp4/2(data_in)
  Counter19/1 -> avg4/1(addr)
  mov_avg4/2(dout_valid) -> Counter19/1, avg4/3(we)
  Convert13/1 -> Reinterpret44/1
  Reinterpret44/1 -> avg4/2(data_in)
  pipeline46/1 -> Register6/3, Register6/1
  [detection4] -> Logical3/5
  control/25(acc_len5) -> [acc_len4]
  control/38(theta5) -> [theta4]
  Reinterpret47/1 -> Concat11/1
  Reinterpret45/1 -> Concat11/2
  Reinterpret46/1 -> Concat11/3
  Reinterpret48/1 -> Concat11/4
  phase_calc/1(dout_valid) -> Counter11/2, rfi_flag/3(we)
  phase_calc/2(dout3) -> Relational5/2, Reinterpret47/1
  phase_calc/3(dout2) -> Relational6/2, Reinterpret45/1
  phase_calc/4(dout1) -> Relational7/2, Reinterpret46/1
  phase_calc/5(dout0) -> Relational8/2, Reinterpret48/1
  Counter11/1 -> rfi_flag/1(addr)
  Concat11/1 -> rfi_flag/2(data_in)
  c_to_ri/1 -> rfi_detection0/1(sig_re)
  c_to_ri/2 -> rfi_detection0/2(sig_im)
  c_to_ri1/1 -> rfi_detection0/3(ref_re)
  c_to_ri1/2 -> rfi_detection0/4(ref_im)
  c_to_ri2/1 -> rfi_detection1/1(sig_re)
  c_to_ri2/2 -> rfi_detection1/2(sig_im)
  c_to_ri3/1 -> rfi_detection1/3(ref_re)
  c_to_ri3/2 -> rfi_detection1/4(ref_im)
  c_to_ri4/2 -> rfi_detection2/2(sig_im)
  c_to_ri4/1 -> rfi_detection2/1(sig_re)
  c_to_ri5/2 -> rfi_detection2/4(ref_im)
  c_to_ri5/1 -> rfi_detection2/3(ref_re)
  c_to_ri6/2 -> rfi_detection3/2(sig_im)
  c_to_ri6/1 -> rfi_detection3/1(sig_re)
  c_to_ri7/1 -> rfi_detection3/3(ref_re)
  c_to_ri7/2 -> rfi_detection3/4(ref_im)
  [beam0] -> c_to_ri/1
  [rfi0] -> c_to_ri1/1
  [beam1] -> c_to_ri2/1
  [rfi1] -> c_to_ri3/1
  [beam2] -> c_to_ri4/1
  [rfi2] -> c_to_ri5/1
  [beam3] -> c_to_ri6/1
  [rfi3] -> c_to_ri7/1
  [rfi_acc_len] -> rfi_detection1/7(acc_len)
  [rfi_acc_len] -> rfi_detection2/7(acc_len)
  [rfi_acc_len] -> rfi_detection3/7(acc_len)
  [rfi_acc_len] -> rfi_detection0/7(acc_len)
  [cnt_rst] -> Register7/2, rfi_detection0/8(cnt_rst)
  [cnt_rst] -> Register8/2, rfi_detection1/8(cnt_rst)
  [cnt_rst] -> Register9/2, rfi_detection2/8(cnt_rst)
  [cnt_rst] -> Register10/2, rfi_detection3/8(cnt_rst)
  Register7/1 -> rfi_detection0/5(din_valid)
  Register8/1 -> rfi_detection1/5(din_valid)
  Register9/1 -> rfi_detection2/5(din_valid)
  Register10/1 -> rfi_detection3/5(din_valid)
  Logical4/1 -> Register7/3, Register7/1
  [rfi_en] -> Logical4/1
  [beam_sync] -> Logical4/2, rfi_detection0/6(sync_in)
  [rfi_en] -> Logical5/1
  [beam_sync] -> rfi_detection1/6(sync_in), Logical5/2
  Logical5/1 -> Register8/3, Register8/1
  [rfi_en] -> Logical6/1
  [beam_sync] -> rfi_detection2/6(sync_in), Logical6/2
  Logical6/1 -> Register9/1, Register9/3
  [rfi_en] -> Logical7/1
  [beam_sync] -> rfi_detection3/6(sync_in), Logical7/2
  Logical7/1 -> Register10/3, Register10/1
  rfi_detection3/1(pow_data) -> [rfi_pow3]
  rfi_detection3/2(corr_data) -> [rfi_corr3]
  rfi_detection2/1(pow_data) -> [rfi_pow2]
  rfi_detection2/2(corr_data) -> [rfi_corr2]
  rfi_detection1/1(pow_data) -> [rfi_pow1]
  rfi_detection1/2(corr_data) -> [rfi_corr1]
  rfi_detection0/1(pow_data) -> [rfi_pow0]
  rfi_detection0/2(corr_data) -> [rfi_corr0]
  rfi_detection3/3(dout_valid) -> [rfi_pow_valid]
  [rfi_pow_valid] -> edge_detect/1, phase_calc/1(rfi_pow_valid)
  [rfi_pow3] -> phase_calc/2(rfi_pow3)
  [rfi_corr3] -> phase_calc/3(rfi_corr3)
  [rfi_pow2] -> phase_calc/4(rfi_pow2)
  [rfi_corr2] -> phase_calc/5(rfi_corr2)
  [rfi_pow1] -> phase_calc/6(rfi_pow1)
  [rfi_corr1] -> phase_calc/7(rfi_corr1)
  [rfi_pow0] -> phase_calc/8(rfi_pow0)
  [rfi_corr0] -> phase_calc/9(rfi_corr0)
  edge_detect/1 -> Counter11/1
  Convert14/1 -> Reinterpret21/1
  Convert15/1 -> Reinterpret22/1
  Convert16/1 -> Reinterpret23/1
  Convert17/1 -> Reinterpret27/1
  Reinterpret22/1 -> Concat7/2
  Reinterpret23/1 -> Concat7/3
  Reinterpret27/1 -> Concat7/4
  Reinterpret21/1 -> Concat7/1
  [rfi_corr3] -> Convert14/1
  [rfi_corr2] -> Convert15/1
  [rfi_corr1] -> Convert16/1
  [rfi_corr0] -> Convert17/1
  Concat7/1 -> rfi_corr/2(data_in)
  [rfi_pow_valid] -> edge_detect1/1, pipeline25/1(d)
  edge_detect1/1 -> Counter10/1
  Convert18/1 -> Reinterpret28/1
  Convert19/1 -> Reinterpret29/1
  Convert20/1 -> Reinterpret30/1
  Convert21/1 -> Reinterpret32/1
  Reinterpret29/1 -> Concat8/2
  Reinterpret30/1 -> Concat8/3
  Reinterpret32/1 -> Concat8/4
  Reinterpret28/1 -> Concat8/1
  [rfi_pow3] -> Convert18/1
  [rfi_pow2] -> Convert19/1
  [rfi_pow1] -> Convert20/1
  [rfi_pow0] -> Convert21/1
  Concat8/1 -> rfi_pow/2(data_in)
  pipeline25/1(q) -> rfi_pow/3(we), rfi_corr/3(we), Counter10/2
  Counter10/1 -> rfi_pow/1(addr), rfi_corr/1(addr)
  control/45(rfi_acc_len) -> [rfi_acc_len]
  control/47(rfi_en) -> [rfi_en]
  control/48(rfi_hold) -> [rfi_hold]
  [rfi_thresh] -> Relational6/1, Relational7/1, Relational8/1, Relational5/1
  Relational5/1 -> Logical8/1
  Relational6/1 -> Logical8/2
  Relational7/1 -> Logical8/3
  Relational8/1 -> Logical8/4
  control/46(rfi_thresh) -> [rfi_thresh]
  Logical8/1 -> Logical10/2, Register11/1, Register11/3
  Register11/1 -> Counter20/2, pipeline13/1
  Counter20/1 -> Relational9/2
  Logical9/1 -> Register11/2
  Relational9/1 -> Logical9/2, Logical10/1
  Logical10/1 -> Counter20/1
  [rfi_hold] -> Relational9/1
  [rfi_en] -> Inverter1/1
  Inverter1/1 -> Logical9/1
  pipeline13/1 -> [rfi_detected]
  Relational/1 -> Logical11/2
  [rfi_detected] -> Inverter2/1
  Logical12/1 -> pipeline41/1
  Relational1/1 -> Logical12/2
  [rfi_detected] -> Inverter4/1
  Logical13/1 -> pipeline40/1
  Relational2/1 -> Logical13/2
  [rfi_detected] -> Inverter5/1
  Logical14/1 -> pipeline39/1
  Relational3/1 -> Logical14/2
  [rfi_detected] -> Inverter6/1
  Logical15/1 -> pipeline46/1
  Relational4/1 -> Logical15/2
  [rfi_detected] -> Inverter7/1
  control/33(en_dedisp) -> [en_dedisp]
  Logical16/1 -> enabled_vacc1/1(new_acc), Register12/3, Register12/1
  acc_cntrl6/1(new_acc) -> Logical16/2
  [en_dedisp] -> Logical16/1
  Register12/1 -> Logical25/1
  [rst_dedisp] -> Register12/2
  Logical17/1 -> Register13/3, Register13/1, enabled_vacc2/1(new_acc)
  acc_cntrl7/1(new_acc) -> Logical17/2
  [en_dedisp] -> Logical17/1
  Register13/1 -> Logical22/1
  [rst_dedisp] -> Register13/2
  Logical18/1 -> enabled_vacc3/1(new_acc), Register14/3, Register14/1
  acc_cntrl8/1(new_acc) -> Logical18/2
  [en_dedisp] -> Logical18/1
  Register14/1 -> Logical20/1
  [rst_dedisp] -> Register14/2
  Logical19/1 -> Register15/3, Register15/1, enabled_vacc4/1(new_acc)
  acc_cntrl9/1(new_acc) -> Logical19/2
  [en_dedisp] -> Logical19/1
  Register15/1 -> Logical21/1
  [rst_dedisp] -> Register15/2
  Logical20/1 -> enabled_vacc3/3(din_valid)
  pipeline38/1(q) -> Logical20/2
  Logical21/1 -> enabled_vacc4/3(din_valid)
  pipeline45/1(q) -> Logical21/2
  Logical22/1 -> enabled_vacc2/3(din_valid)
  pipeline36/1(q) -> Logical22/2
  Logical25/1 -> enabled_vacc1/3(din_valid)
  pipeline34/1(q) -> Logical25/2
  Logical26/1 -> enabled_vacc0/3(din_valid)
  pipeline16/1(q) -> Logical26/2
  acc_cntrl5/1(new_acc) -> Logical27/2
  [en_dedisp] -> Logical27/1
  [rst_dedisp] -> Register16/2
  Register16/1 -> Logical26/1
  Inverter2/1 -> Logical11/1
  Inverter4/1 -> Logical12/1
  Inverter5/1 -> Logical13/1
  Inverter6/1 -> Logical14/1
  Inverter7/1 -> Logical15/1
  [acc_len5] -> acc_cntrl10/1(acc_len)
  [sd0] -> acc_cntrl10/2(sync)
  [cnt_rst] -> acc_cntrl10/3(rst)
  pipeline14/1(q) -> enabled_vacc5/2(din)
  [m0e5] -> pipeline26/1(d)
  [m0d5] -> pipeline14/1(d)
  enabled_vacc5/1(dout) -> pre_dedisp_conv5/1(din)
  enabled_vacc5/2(dout_valid) -> pre_dedisp_conv5/2(din_valid)
  pre_dedisp_conv5/2(dout_valid) -> pre_dedisp_delay5/2(din_valid)
  pre_dedisp_conv5/1(dout) -> pre_dedisp_delay5/1(In1)
  pre_dedisp_delay5/2(dout_valid) -> dedispersor5/3(din_valid)
  pre_dedisp_delay5/1(Out1) -> dedispersor5/2(din)
  [rst_dedisp] -> dedispersor5/1(rst)
  dedispersor5/1(integ_pow) -> post_dedisp_conv5/1(din)
  dedispersor5/2(integ_valid) -> post_dedisp_conv5/2(din_valid)
  post_dedisp_conv5/1(dout) -> post_dedisp_delay5/1(In1)
  post_dedisp_conv5/2(dout_valid) -> post_dedisp_delay5/2(din_valid)
  post_dedisp_delay5/1(Out1) -> Convert1/1, Relational10/1, mov_avg5/2(din)
  [rst_dedisp] -> mov_avg5/1(rst)
  mov_avg5/1(dout) -> add_stat5/2
  add_stat5/1 -> Relational10/2, Convert22/1
  [theta5] -> add_stat5/1
  [rst_detection] -> Register18/2
  Register18/1 -> [detection5]
  Counter21/1 -> dedisp5/1(addr)
  post_dedisp_delay5/2(dout_valid) -> Counter21/1, dedisp5/3(we), mov_avg5/3(din_valid)
  Convert1/1 -> Reinterpret18/1
  Reinterpret18/1 -> dedisp5/2(data_in)
  Counter22/1 -> avg5/1(addr)
  mov_avg5/2(dout_valid) -> Counter22/1, avg5/3(we)
  Convert22/1 -> Reinterpret33/1
  Reinterpret33/1 -> avg5/2(data_in)
  pipeline28/1 -> Register18/3, Register18/1
  Logical28/1 -> pipeline28/1
  Relational10/1 -> Logical28/2
  [rfi_detected] -> Inverter8/1
  Logical29/1 -> Register17/3, Register17/1, enabled_vacc5/1(new_acc)
  acc_cntrl10/1(new_acc) -> Logical29/2
  [en_dedisp] -> Logical29/1
  Register17/1 -> Logical30/1
  [rst_dedisp] -> Register17/2
  Logical30/1 -> enabled_vacc5/3(din_valid)
  pipeline26/1(q) -> Logical30/2
  Inverter8/1 -> Logical28/1
  [detection5] -> Logical3/6
  control/26(acc_len6) -> [acc_len5]
  control/39(theta6) -> [theta5]
  pipeline298/1 -> bus_expand/1(bus_in)
  Constant4/1 -> snapshot/2(we), snapshot/3(trig)
  bus_expand/1(msb_out8) -> Convert25/1
  bus_expand/2(out7) -> Convert26/1
  bus_expand/3(out6) -> Convert27/1
  bus_expand/4(out5) -> Convert28/1
  bus_expand/5(out4) -> Convert29/1
  bus_expand/6(out3) -> Convert30/1
  bus_expand/7(out2) -> Convert23/1
  bus_expand/8(lsb_out1) -> Convert24/1
  Convert24/1 -> bus_create4/8(in8)
  Convert23/1 -> bus_create4/7(in7)
  Convert30/1 -> bus_create4/6(in6)
  Convert29/1 -> bus_create4/5(in5)
  Convert28/1 -> bus_create4/4(in4)
  Convert27/1 -> bus_create4/3(in3)
  Convert26/1 -> bus_create4/2(in2)
  Convert25/1 -> bus_create4/1(in1)
  bus_create4/1(bus_out) -> pipeline29/1
  [adc0] -> pipeline298/1
  pipeline29/1 -> snapshot/1(din)
  [acc_len6] -> acc_cntrl11/1(acc_len)
  [sd0] -> acc_cntrl11/2(sync)
  [cnt_rst] -> acc_cntrl11/3(rst)
  pipeline31/1(q) -> enabled_vacc6/2(din)
  [m0e6] -> pipeline32/1(d)
  [m0d6] -> pipeline31/1(d)
  enabled_vacc6/1(dout) -> pre_dedisp_conv6/1(din)
  enabled_vacc6/2(dout_valid) -> pre_dedisp_conv6/2(din_valid)
  pre_dedisp_conv6/2(dout_valid) -> pre_dedisp_delay6/2(din_valid)
  pre_dedisp_conv6/1(dout) -> pre_dedisp_delay6/1(In1)
  pre_dedisp_delay6/2(dout_valid) -> dedispersor6/3(din_valid)
  pre_dedisp_delay6/1(Out1) -> dedispersor6/2(din)
  [rst_dedisp] -> dedispersor6/1(rst)
  dedispersor6/1(integ_pow) -> post_dedisp_conv6/1(din)
  dedispersor6/2(integ_valid) -> post_dedisp_conv6/2(din_valid)
  post_dedisp_conv6/1(dout) -> post_dedisp_delay6/1(In1)
  post_dedisp_conv6/2(dout_valid) -> post_dedisp_delay6/2(din_valid)
  post_dedisp_delay6/1(Out1) -> Convert31/1, Relational11/1, mov_avg6/2(din)
  [rst_dedisp] -> mov_avg6/1(rst)
  mov_avg6/1(dout) -> add_stat6/2
  add_stat6/1 -> Relational11/2, Convert32/1
  [theta6] -> add_stat6/1
  [rst_detection] -> Register20/2
  Register20/1 -> [detection6]
  Counter23/1 -> dedisp6/1(addr)
  post_dedisp_delay6/2(dout_valid) -> Counter23/1, dedisp6/3(we), mov_avg6/3(din_valid)
  Convert31/1 -> Reinterpret34/1
  Reinterpret34/1 -> dedisp6/2(data_in)
  Counter24/1 -> avg6/1(addr)
  mov_avg6/2(dout_valid) -> Counter24/1, avg6/3(we)
  Convert32/1 -> Reinterpret39/1
  Reinterpret39/1 -> avg6/2(data_in)
  pipeline47/1 -> Register20/3, Register20/1
  Logical31/1 -> pipeline47/1
  Relational11/1 -> Logical31/2
  [rfi_detected] -> Inverter9/1
  Logical32/1 -> Register19/3, Register19/1, enabled_vacc6/1(new_acc)
  acc_cntrl11/1(new_acc) -> Logical32/2
  [en_dedisp] -> Logical32/1
  Register19/1 -> Logical33/1
  [rst_dedisp] -> Register19/2
  Logical33/1 -> enabled_vacc6/3(din_valid)
  pipeline32/1(q) -> Logical33/2
  Inverter9/1 -> Logical31/1
  [detection6] -> Logical3/7
  control/27(acc_len7) -> [acc_len6]
  control/40(theta7) -> [theta6]
  beam_power/3(dout1) -> post_flag_delay1/3(In2)
  beam_power/4(dout2) -> post_flag_delay1/4(In3)
  beam_power/2(dout0) -> post_flag_delay1/2(In1)
  beam_power/5(dout3) -> post_flag_delay1/5(In4)
  post_flag_delay1/4(Out3) -> beam_power_conv/4(In3)
  post_flag_delay1/2(Out1) -> beam_power_conv/2(In1)
  post_flag_delay1/3(Out2) -> beam_power_conv/3(In2)
  post_flag_delay1/1(sync_out) -> beam_power_conv/1(sync_in)
  post_flag_delay1/5(Out4) -> beam_power_conv/5(In4)
  [acc_len7] -> acc_cntrl12/1(acc_len)
  [sd0] -> acc_cntrl12/2(sync)
  [cnt_rst] -> acc_cntrl12/3(rst)
  pipeline48/1(q) -> enabled_vacc7/2(din)
  [m0e7] -> pipeline51/1(d)
  [m0d7] -> pipeline48/1(d)
  enabled_vacc7/1(dout) -> pre_dedisp_conv7/1(din)
  enabled_vacc7/2(dout_valid) -> pre_dedisp_conv7/2(din_valid)
  pre_dedisp_conv7/2(dout_valid) -> pre_dedisp_delay7/2(din_valid)
  pre_dedisp_conv7/1(dout) -> pre_dedisp_delay7/1(In1)
  pre_dedisp_delay7/2(dout_valid) -> dedispersor7/3(din_valid)
  pre_dedisp_delay7/1(Out1) -> dedispersor7/2(din)
  [rst_dedisp] -> dedispersor7/1(rst)
  dedispersor7/1(integ_pow) -> post_dedisp_conv7/1(din)
  dedispersor7/2(integ_valid) -> post_dedisp_conv7/2(din_valid)
  post_dedisp_conv7/1(dout) -> post_dedisp_delay7/1(In1)
  post_dedisp_conv7/2(dout_valid) -> post_dedisp_delay7/2(din_valid)
  post_dedisp_delay7/1(Out1) -> Convert33/1, Relational12/1, mov_avg7/2(din)
  [rst_dedisp] -> mov_avg7/1(rst)
  mov_avg7/1(dout) -> add_stat7/2
  add_stat7/1 -> Relational12/2, Convert34/1
  [theta7] -> add_stat7/1
  [rst_detection] -> Register22/2
  Register22/1 -> [detection7]
  Counter25/1 -> dedisp7/1(addr)
  post_dedisp_delay7/2(dout_valid) -> Counter25/1, dedisp7/3(we), mov_avg7/3(din_valid)
  Convert33/1 -> Reinterpret42/1
  Reinterpret42/1 -> dedisp7/2(data_in)
  Counter26/1 -> avg7/1(addr)
  mov_avg7/2(dout_valid) -> Counter26/1, avg7/3(we)
  Convert34/1 -> Reinterpret49/1
  Reinterpret49/1 -> avg7/2(data_in)
  pipeline54/1 -> Register22/3, Register22/1
  Logical34/1 -> pipeline54/1
  Relational12/1 -> Logical34/2
  [rfi_detected] -> Inverter10/1
  Logical35/1 -> Register21/3, Register21/1, enabled_vacc7/1(new_acc)
  acc_cntrl12/1(new_acc) -> Logical35/2
  [en_dedisp] -> Logical35/1
  Register21/1 -> Logical36/1
  [rst_dedisp] -> Register21/2
  Logical36/1 -> enabled_vacc7/3(din_valid)
  pipeline51/1(q) -> Logical36/2
  Inverter10/1 -> Logical34/1
  control/41(theta8) -> [theta7]
  control/28(acc_len8) -> [acc_len7]
  [detection7] -> Logical3/8
  [acc_len8] -> acc_cntrl13/1(acc_len)
  [sd0] -> acc_cntrl13/2(sync)
  [cnt_rst] -> acc_cntrl13/3(rst)
  pipeline56/1(q) -> enabled_vacc8/2(din)
  [m0e8] -> pipeline57/1(d)
  [m0d8] -> pipeline56/1(d)
  enabled_vacc8/1(dout) -> pre_dedisp_conv8/1(din)
  enabled_vacc8/2(dout_valid) -> pre_dedisp_conv8/2(din_valid)
  pre_dedisp_conv8/2(dout_valid) -> pre_dedisp_delay8/2(din_valid)
  pre_dedisp_conv8/1(dout) -> pre_dedisp_delay8/1(In1)
  pre_dedisp_delay8/2(dout_valid) -> dedispersor8/3(din_valid)
  pre_dedisp_delay8/1(Out1) -> dedispersor8/2(din)
  [rst_dedisp] -> dedispersor8/1(rst)
  dedispersor8/1(integ_pow) -> post_dedisp_conv8/1(din)
  dedispersor8/2(integ_valid) -> post_dedisp_conv8/2(din_valid)
  post_dedisp_conv8/1(dout) -> post_dedisp_delay8/1(In1)
  post_dedisp_conv8/2(dout_valid) -> post_dedisp_delay8/2(din_valid)
  post_dedisp_delay8/1(Out1) -> Convert35/1, Relational13/1, mov_avg8/2(din)
  [rst_dedisp] -> mov_avg8/1(rst)
  mov_avg8/1(dout) -> add_stat8/2
  add_stat8/1 -> Relational13/2, Convert36/1
  [theta8] -> add_stat8/1
  [rst_detection] -> Register24/2
  Register24/1 -> [detection8]
  Counter27/1 -> dedisp8/1(addr)
  post_dedisp_delay8/2(dout_valid) -> Counter27/1, dedisp8/3(we), mov_avg8/3(din_valid)
  Convert35/1 -> Reinterpret50/1
  Reinterpret50/1 -> dedisp8/2(data_in)
  Counter28/1 -> avg8/1(addr)
  mov_avg8/2(dout_valid) -> Counter28/1, avg8/3(we)
  Convert36/1 -> Reinterpret51/1
  Reinterpret51/1 -> avg8/2(data_in)
  pipeline61/1 -> Register24/3, Register24/1
  Logical37/1 -> pipeline61/1
  Relational13/1 -> Logical37/2
  [rfi_detected] -> Inverter11/1
  Logical38/1 -> Register23/3, Register23/1, enabled_vacc8/1(new_acc)
  acc_cntrl13/1(new_acc) -> Logical38/2
  [en_dedisp] -> Logical38/1
  Register23/1 -> Logical39/1
  [rst_dedisp] -> Register23/2
  Logical39/1 -> enabled_vacc8/3(din_valid)
  pipeline57/1(q) -> Logical39/2
  Inverter11/1 -> Logical37/1
  [detection8] -> Logical3/9
  control/29(acc_len9) -> [acc_len8]
  control/42(theta9) -> [theta8]
  [acc_len9] -> acc_cntrl14/1(acc_len)
  [sd0] -> acc_cntrl14/2(sync)
  [cnt_rst] -> acc_cntrl14/3(rst)
  pipeline62/1(q) -> enabled_vacc9/2(din)
  [m0e9] -> pipeline65/1(d)
  [m0d9] -> pipeline62/1(d)
  enabled_vacc9/1(dout) -> pre_dedisp_conv9/1(din)
  enabled_vacc9/2(dout_valid) -> pre_dedisp_conv9/2(din_valid)
  pre_dedisp_conv9/2(dout_valid) -> pre_dedisp_delay9/2(din_valid)
  pre_dedisp_conv9/1(dout) -> pre_dedisp_delay9/1(In1)
  pre_dedisp_delay9/2(dout_valid) -> dedispersor9/3(din_valid)
  pre_dedisp_delay9/1(Out1) -> dedispersor9/2(din)
  [rst_dedisp] -> dedispersor9/1(rst)
  dedispersor9/1(integ_pow) -> post_dedisp_conv9/1(din)
  dedispersor9/2(integ_valid) -> post_dedisp_conv9/2(din_valid)
  post_dedisp_conv9/1(dout) -> post_dedisp_delay9/1(In1)
  post_dedisp_conv9/2(dout_valid) -> post_dedisp_delay9/2(din_valid)
  post_dedisp_delay9/1(Out1) -> Convert37/1, Relational14/1, mov_avg9/2(din)
  [rst_dedisp] -> mov_avg9/1(rst)
  mov_avg9/1(dout) -> add_stat9/2
  add_stat9/1 -> Relational14/2, Convert38/1
  [theta9] -> add_stat9/1
  [rst_detection] -> Register26/2
  Register26/1 -> [detection9]
  Counter29/1 -> dedisp9/1(addr)
  post_dedisp_delay9/2(dout_valid) -> mov_avg9/3(din_valid), Counter29/1, dedisp9/3(we)
  Convert37/1 -> Reinterpret52/1
  Reinterpret52/1 -> dedisp9/2(data_in)
  Counter30/1 -> avg9/1(addr)
  mov_avg9/2(dout_valid) -> Counter30/1, avg9/3(we)
  Convert38/1 -> Reinterpret53/1
  Reinterpret53/1 -> avg9/2(data_in)
  pipeline66/1 -> Register26/3, Register26/1
  Logical40/1 -> pipeline66/1
  Relational14/1 -> Logical40/2
  [rfi_detected] -> Inverter12/1
  Logical41/1 -> Register25/3, Register25/1, enabled_vacc9/1(new_acc)
  acc_cntrl14/1(new_acc) -> Logical41/2
  [en_dedisp] -> Logical41/1
  Register25/1 -> Logical42/1
  [rst_dedisp] -> Register25/2
  Logical42/1 -> enabled_vacc9/3(din_valid)
  pipeline65/1(q) -> Logical42/2
  Inverter12/1 -> Logical40/1
  [detection9] -> Logical3/10
  control/30(acc_len10) -> [acc_len9]
  control/43(theta10) -> [theta9]
  Concat9/1 -> pipeline69/1
  pipeline69/1 -> control/1(frb_detection)
  [rfi_detected] -> control/2(rfi_detected)
  [acc_len10] -> acc_cntrl15/1(acc_len)
  [sd0] -> acc_cntrl15/2(sync)
  [cnt_rst] -> acc_cntrl15/3(rst)
  pipeline70/1(q) -> enabled_vacc10/2(din)
  [m0e10] -> pipeline72/1(d)
  [m0d10] -> pipeline70/1(d)
  enabled_vacc10/1(dout) -> pre_dedisp_conv10/1(din)
  enabled_vacc10/2(dout_valid) -> pre_dedisp_conv10/2(din_valid)
  pre_dedisp_conv10/2(dout_valid) -> pre_dedisp_delay10/2(din_valid)
  pre_dedisp_conv10/1(dout) -> pre_dedisp_delay10/1(In1)
  pre_dedisp_delay10/2(dout_valid) -> dedispersor10/3(din_valid)
  pre_dedisp_delay10/1(Out1) -> dedispersor10/2(din)
  [rst_dedisp] -> dedispersor10/1(rst)
  dedispersor10/1(integ_pow) -> post_dedisp_conv10/1(din)
  dedispersor10/2(integ_valid) -> post_dedisp_conv10/2(din_valid)
  post_dedisp_conv10/1(dout) -> post_dedisp_delay10/1(In1)
  post_dedisp_conv10/2(dout_valid) -> post_dedisp_delay10/2(din_valid)
  post_dedisp_delay10/1(Out1) -> Convert39/1, Relational15/1, mov_avg10/2(din)
  [rst_dedisp] -> mov_avg10/1(rst)
  mov_avg10/1(dout) -> add_stat10/2
  add_stat10/1 -> Relational15/2, Convert40/1
  [theta10] -> add_stat10/1
  [rst_detection] -> Register28/2
  Register28/1 -> [detection10]
  Counter31/1 -> dedisp10/1(addr)
  post_dedisp_delay10/2(dout_valid) -> mov_avg10/3(din_valid), Counter31/1, dedisp10/3(we)
  Convert39/1 -> Reinterpret54/1
  Reinterpret54/1 -> dedisp10/2(data_in)
  Counter32/1 -> avg10/1(addr)
  mov_avg10/2(dout_valid) -> Counter32/1, avg10/3(we)
  Convert40/1 -> Reinterpret55/1
  Reinterpret55/1 -> avg10/2(data_in)
  pipeline74/1 -> Register28/3, Register28/1
  Logical43/1 -> pipeline74/1
  Relational15/1 -> Logical43/2
  [rfi_detected] -> Inverter13/1
  Logical44/1 -> Register27/3, Register27/1, enabled_vacc10/1(new_acc)
  acc_cntrl15/1(new_acc) -> Logical44/2
  [en_dedisp] -> Logical44/1
  Register27/1 -> Logical45/1
  [rst_dedisp] -> Register27/2
  Logical45/1 -> enabled_vacc10/3(din_valid)
  pipeline72/1(q) -> Logical45/2
  Inverter13/1 -> Logical43/1
  [detection10] -> Logical3/11
  control/31(acc_len11) -> [acc_len10]
  control/44(theta11) -> [theta10]
  [detection9] -> Concat9/2
  [detection8] -> Concat9/3
  [detection7] -> Concat9/4
  [detection6] -> Concat9/5
  [detection5] -> Concat9/6
  [detection4] -> Concat9/7
  [detection3] -> Concat9/8
  [detection2] -> Concat9/9
  [detection1] -> Concat9/10
  [detection0] -> Concat9/11
  [detection10] -> Concat9/1
